simulink model "SPGF_FSK_0000_R2022b"  (R2022b)
settings: Solver=ode4  StartTime=0.0  StopTime=1.4  FixedStep=50e-6/50  RelTol=1e-3  EnableMultiTasking=on
undefined symbols (not defined in the file): D11, Delta
libraries: spsSeriesRLCBranchLib x1646, spsGroundLib x360, spsStairGeneratorLib x147, spsIdealSwitchLib x145, spsCurrentMeasurementLib x145, spsUniversalBridgeLib x76, spsThreePhaseSeriesRLCLoadLib x57, simulink x45, spsBistableLib x36, spsSequenceAnalyzerLib x31, spsThreePhaseParallelRLCLoadLib x20, spsThreePhaseTransformerTwoWindingsLib x20
(part 20 of 40)

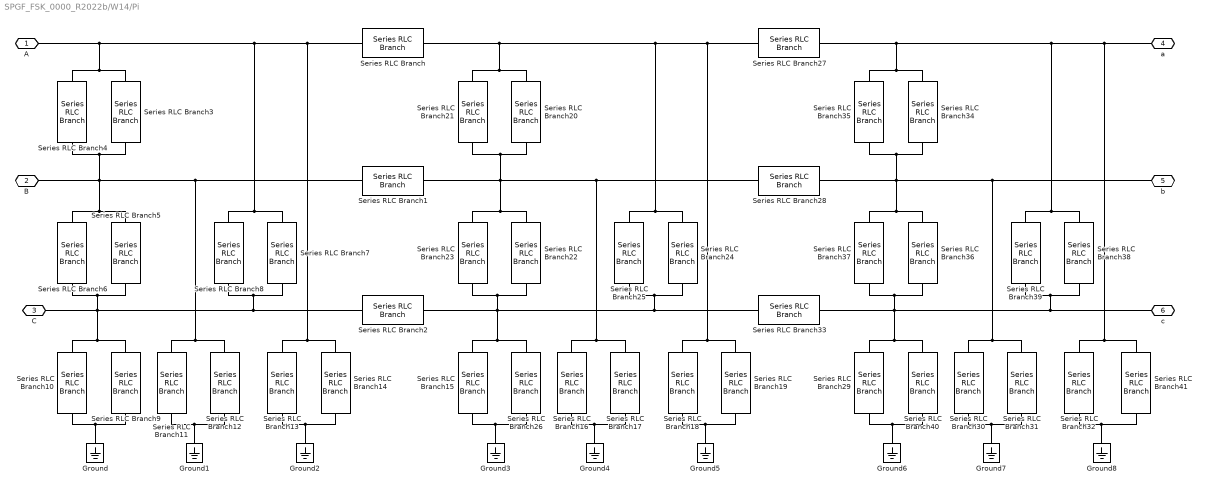
== system SPGF_FSK_0000_R2022b/W14/Pi ==
  Ground{,1..8} (9 alike) : spsGroundLib/Ground  LConnTagsString=a
  Series RLC Branch{,1..2,27..28,33} (6 alike) : spsSeriesRLCBranchLib/Series RLC Branch  LConnTagsString=__new0  RConnTagsString=__new0  BranchType=RL  Resistance=R/2  Inductance=L/2  SetiL0=off  InitialCurrent=0  Capacitance=1e-6  Setx0=off  InitialVoltage=0  Measurements=None
  Series RLC Branch{10..11,13,29..30,32} (6 alike) : spsSeriesRLCBranchLib/Series RLC Branch  LConnTagsString=__new0  RConnTagsString=__new0  BranchType=R  Resistance=Rfg*4  Inductance=L/2  SetiL0=off  InitialCurrent=0  Capacitance=1e-6  Setx0=off  InitialVoltage=0  Measurements=None
  Series RLC Branch{9,12,14,31,40..41} (6 alike) : spsSeriesRLCBranchLib/Series RLC Branch  LConnTagsString=__new0  RConnTagsString=__new0  BranchType=C  Resistance=R/2  Inductance=L/2  SetiL0=off  InitialCurrent=0  Capacitance=Cfg*0.25  Setx0=off  InitialVoltage=0  Measurements=None
  Series RLC Branch15 : spsSeriesRLCBranchLib/Series RLC Branch  LConnTagsString=__new0  RConnTagsString=__new0  BranchType=R  Resistance=Rfg*2  Inductance=L/2  SetiL0=off  InitialCurrent=0  Capacitance=1e-6  Setx0=off  InitialVoltage=0  Measurements=None
  Series RLC Branch16 : spsSeriesRLCBranchLib/Series RLC Branch  LConnTagsString=__new0  RConnTagsString=__new0  BranchType=R  Resistance=Rfg*2  Inductance=L/2  SetiL0=off  InitialCurrent=0  Capacitance=1e-6  Setx0=off  InitialVoltage=0  Measurements=None
  Series RLC Branch17 : spsSeriesRLCBranchLib/Series RLC Branch  LConnTagsString=__new0  RConnTagsString=__new0  BranchType=C  Resistance=R/2  Inductance=L/2  SetiL0=off  InitialCurrent=0  Capacitance=Cfg*0.5  Setx0=off  InitialVoltage=0  Measurements=None
  Series RLC Branch18 : spsSeriesRLCBranchLib/Series RLC Branch  LConnTagsString=__new0  RConnTagsString=__new0  BranchType=R  Resistance=Rfg*2  Inductance=L/2  SetiL0=off  InitialCurrent=0  Capacitance=1e-6  Setx0=off  InitialVoltage=0  Measurements=None
  Series RLC Branch19 : spsSeriesRLCBranchLib/Series RLC Branch  LConnTagsString=__new0  RConnTagsString=__new0  BranchType=C  Resistance=R/2  Inductance=L/2  SetiL0=off  InitialCurrent=0  Capacitance=Cfg*0.5  Setx0=off  InitialVoltage=0  Measurements=None
  Series RLC Branch20 : spsSeriesRLCBranchLib/Series RLC Branch  LConnTagsString=__new0  RConnTagsString=__new0  BranchType=C  Resistance=R/2  Inductance=L/2  SetiL0=off  InitialCurrent=0  Capacitance=Cmf*0.5  Setx0=off  InitialVoltage=0  Measurements=None
  Series RLC Branch21 : spsSeriesRLCBranchLib/Series RLC Branch  LConnTagsString=__new0  RConnTagsString=__new0  BranchType=R  Resistance=Rmf*2  Inductance=L/2  SetiL0=off  InitialCurrent=0  Capacitance=1e-6  Setx0=off  InitialVoltage=0  Measurements=None
  Series RLC Branch22 : spsSeriesRLCBranchLib/Series RLC Branch  LConnTagsString=__new0  RConnTagsString=__new0  BranchType=C  Resistance=R/2  Inductance=L/2  SetiL0=off  InitialCurrent=0  Capacitance=Cmf*0.5  Setx0=off  InitialVoltage=0  Measurements=None
  Series RLC Branch23 : spsSeriesRLCBranchLib/Series RLC Branch  LConnTagsString=__new0  RConnTagsString=__new0  BranchType=R  Resistance=Rmf*2  Inductance=L/2  SetiL0=off  InitialCurrent=0  Capacitance=1e-6  Setx0=off  InitialVoltage=0  Measurements=None
  Series RLC Branch24 : spsSeriesRLCBranchLib/Series RLC Branch  LConnTagsString=__new0  RConnTagsString=__new0  BranchType=C  Resistance=R/2  Inductance=L/2  SetiL0=off  InitialCurrent=0  Capacitance=Cmf*0.5  Setx0=off  InitialVoltage=0  Measurements=None
  Series RLC Branch25 : spsSeriesRLCBranchLib/Series RLC Branch  LConnTagsString=__new0  RConnTagsString=__new0  BranchType=R  Resistance=Rmf*2  Inductance=L/2  SetiL0=off  InitialCurrent=0  Capacitance=1e-6  Setx0=off  InitialVoltage=0  Measurements=None
  Series RLC Branch26 : spsSeriesRLCBranchLib/Series RLC Branch  LConnTagsString=__new0  RConnTagsString=__new0  BranchType=C  Resistance=R/2  Inductance=L/2  SetiL0=off  InitialCurrent=0  Capacitance=Cfg*0.5  Setx0=off  InitialVoltage=0  Measurements=None
  Series RLC Branch{3,5,7,34,36,38} (6 alike) : spsSeriesRLCBranchLib/Series RLC Branch  LConnTagsString=__new0  RConnTagsString=__new0  BranchType=C  Resistance=R/2  Inductance=L/2  SetiL0=off  InitialCurrent=0  Capacitance=Cmf*0.25  Setx0=off  InitialVoltage=0  Measurements=None
  Series RLC Branch{4,6,8,35,37,39} (6 alike) : spsSeriesRLCBranchLib/Series RLC Branch  LConnTagsString=__new0  RConnTagsString=__new0  BranchType=R  Resistance=Rmf*4  Inductance=L/2  SetiL0=off  InitialCurrent=0  Capacitance=1e-6  Setx0=off  InitialVoltage=0  Measurements=None
  A : PMIOPort  Side=Left
  B : PMIOPort  Port=2  Side=Left
  C : PMIOPort  Port=3  Side=Left
  a : PMIOPort  Port=4  Side=Right
  b : PMIOPort  Port=5  Side=Right
  c : PMIOPort  Port=6  Side=Right
  connections:
  Ground8/LConn1 -- Series RLC Branch41/RConn1 -- Series RLC Branch32/RConn1
  Ground7/LConn1 -- Series RLC Branch30/RConn1 -- Series RLC Branch31/RConn1
  Ground6/LConn1 -- Series RLC Branch40/RConn1 -- Series RLC Branch29/RConn1
  Series RLC Branch40/LConn1 -- Series RLC Branch33/RConn1 -- Series RLC Branch38/RConn1 -- Series RLC Branch39/RConn1 -- c/RConn1 -- Series RLC Branch37/RConn1 -- Series RLC Branch36/RConn1 -- Series RLC Branch29/LConn1
  Series RLC Branch35/LConn1 -- Series RLC Branch27/RConn1 -- Series RLC Branch39/LConn1 -- Series RLC Branch38/LConn1 -- Series RLC Branch32/LConn1 -- Series RLC Branch41/LConn1 -- a/RConn1 -- Series RLC Branch34/LConn1
  Series RLC Branch30/LConn1 -- Series RLC Branch28/RConn1 -- Series RLC Branch37/LConn1 -- Series RLC Branch36/LConn1 -- Series RLC Branch34/RConn1 -- Series RLC Branch35/RConn1 -- b/RConn1 -- Series RLC Branch31/LConn1
  Series RLC Branch19/RConn1 -- Series RLC Branch18/RConn1 -- Ground5/LConn1
  Series RLC Branch16/RConn1 -- Series RLC Branch17/RConn1 -- Ground4/LConn1
  Ground3/LConn1 -- Series RLC Branch15/RConn1 -- Series RLC Branch26/RConn1
  Series RLC Branch23/RConn1 -- Series RLC Branch22/RConn1 -- Series RLC Branch24/RConn1 -- Series RLC Branch25/RConn1 -- Series RLC Branch33/LConn1 -- Series RLC Branch2/RConn1 -- Series RLC Branch15/LConn1 -- Series RLC Branch26/LConn1
  Series RLC Branch25/LConn1 -- Series RLC Branch24/LConn1 -- Series RLC Branch18/LConn1 -- Series RLC Branch19/LConn1 -- Series RLC Branch27/LConn1 -- Series RLC Branch/RConn1 -- Series RLC Branch20/LConn1 -- Series RLC Branch21/LConn1
  Series RLC Branch21/RConn1 -- Series RLC Branch20/RConn1 -- Series RLC Branch22/LConn1 -- Series RLC Branch23/LConn1 -- Series RLC Branch1/RConn1 -- Series RLC Branch28/LConn1 -- Series RLC Branch16/LConn1 -- Series RLC Branch17/LConn1
  Ground2/LConn1 -- Series RLC Branch14/RConn1 -- Series RLC Branch13/RConn1
  Ground1/LConn1 -- Series RLC Branch11/RConn1 -- Series RLC Branch12/RConn1
  Series RLC Branch10/RConn1 -- Ground/LConn1 -- Series RLC Branch9/RConn1
  Series RLC Branch10/LConn1 -- Series RLC Branch6/RConn1 -- Series RLC Branch5/RConn1 -- C/RConn1 -- Series RLC Branch7/RConn1 -- Series RLC Branch8/RConn1 -- Series RLC Branch2/LConn1 -- Series RLC Branch9/LConn1
  Series RLC Branch14/LConn1 -- Series RLC Branch/LConn1 -- Series RLC Branch8/LConn1 -- Series RLC Branch7/LConn1 -- Series RLC Branch3/LConn1 -- Series RLC Branch4/LConn1 -- A/RConn1 -- Series RLC Branch13/LConn1
  Series RLC Branch1/LConn1 -- Series RLC Branch3/RConn1 -- Series RLC Branch4/RConn1 -- B/RConn1 -- Series RLC Branch6/LConn1 -- Series RLC Branch5/LConn1 -- Series RLC Branch11/LConn1 -- Series RLC Branch12/LConn1

== system SPGF_FSK_0000_R2022b/W14/Q ==
  breaker : Subsystem  Commented=on  mask{SwitchA=off, SwitchB=off, SwitchC=off, InitialStatus=[1 1 1], BreakerResistance=0.0001, SnubberResistance=1e6, SnubberCapacitance=inf, TransitionTimes=[0.5 0.7], ShiftTimes=[0 0 0]}
      mask prompts: SwitchA "Switching of phase A"; SwitchB "Switching of phase B"; SwitchC "Switching of phase C"; InitialStatus "Initial status of phase breaker [A, B, C]"; BreakerResistance "Breaker resistance Ron (ohms) :"; SnubberResistance "Snubbers resistance Rp (ohms) :"; SnubberCapacitance "Snubbers capacitance Cp (F) :"; TransitionTimes "Transition times (s) :"; ShiftTimes "Time differences for switch [tA, tB, tC] (s) :"
      mask init: same as SPGF_FSK_0000_R2022b/Feed/Q/breaker
      mask Display:
      | % port_label('input',1,'Iabc');
      | 
      | port_label('lconn',1,'A');
      | port_label('lconn',2,'B');
      | port_label('lconn',3,'C');
      | 
      | port_label('rconn',1,'a');
      | port_label('rconn',2,'b');
      | port_label('rconn',3,'c');
      | 
      | disp('   Q    ');
  meas : Subsystem
  shunt : Subsystem
  A : PMIOPort  Side=Right
  B : PMIOPort  Port=2  Side=Right
  C : PMIOPort  Port=3  Side=Right
  a : PMIOPort  Port=4  Side=Left
  b : PMIOPort  Port=5  Side=Left
  c : PMIOPort  Port=6  Side=Left
  connections:
  shunt/LConn3 -- C/RConn1 -- breaker/LConn3
  shunt/LConn2 -- B/RConn1 -- breaker/LConn2
  A/RConn1 -- shunt/LConn1 -- breaker/LConn1
  meas/RConn1 -- a/RConn1
  meas/RConn2 -- b/RConn1
  meas/RConn3 -- c/RConn1
  meas/LConn3 -- breaker/RConn3 -- shunt/RConn3
  meas/LConn2 -- breaker/RConn2 -- shunt/RConn2
  meas/LConn1 -- breaker/RConn1 -- shunt/RConn1

== system SPGF_FSK_0000_R2022b/W14/concentrated ==
  Ccs/1 : spsSeriesRLCBranchLib/Series RLC Branch  LConnTagsString=__new0  RConnTagsString=__new0  BranchType=C  Resistance=190  Inductance=1e-3  SetiL0=off  InitialCurrent=0  Capacitance=-C_matrix(1,2)/2  Setx0=off  InitialVoltage=0  Measurements=None
  Ccs/2 : spsSeriesRLCBranchLib/Series RLC Branch  LConnTagsString=__new0  RConnTagsString=__new0  BranchType=C  Resistance=190  Inductance=1e-3  SetiL0=off  InitialCurrent=0  Capacitance=-C_matrix(1,2)/2  Setx0=off  InitialVoltage=0  Measurements=None
  Ccs2/1 : spsSeriesRLCBranchLib/Series RLC Branch  LConnTagsString=__new0  RConnTagsString=__new0  BranchType=C  Resistance=190  Inductance=1e-3  SetiL0=off  InitialCurrent=0  Capacitance=-C_matrix(3,4)/2  Setx0=off  InitialVoltage=0  Measurements=None
  Ccs2/2 : spsSeriesRLCBranchLib/Series RLC Branch  LConnTagsString=__new0  RConnTagsString=__new0  BranchType=C  Resistance=190  Inductance=1e-3  SetiL0=off  InitialCurrent=0  Capacitance=-C_matrix(3,4)/2  Setx0=off  InitialVoltage=0  Measurements=None
  Ccs2/3 : spsSeriesRLCBranchLib/Series RLC Branch  LConnTagsString=__new0  RConnTagsString=__new0  BranchType=R  Resistance=-Rg_matrix(3,4)*2  Inductance=1e-3  SetiL0=off  InitialCurrent=0  Capacitance=Rg_matrix(3,4)*2  Setx0=off  InitialVoltage=0  Measurements=None
  Ccs2/4 : spsSeriesRLCBranchLib/Series RLC Branch  LConnTagsString=__new0  RConnTagsString=__new0  BranchType=R  Resistance=-Rg_matrix(3,4)*2  Inductance=1e-3  SetiL0=off  InitialCurrent=0  Capacitance=Rg_matrix(3,4)*2  Setx0=off  InitialVoltage=0  Measurements=None
  Ccs3/1 : spsSeriesRLCBranchLib/Series RLC Branch  LConnTagsString=__new0  RConnTagsString=__new0  BranchType=C  Resistance=190  Inductance=1e-3  SetiL0=off  InitialCurrent=0  Capacitance=-C_matrix(5,6)/2  Setx0=off  InitialVoltage=0  Measurements=None
  Ccs3/2 : spsSeriesRLCBranchLib/Series RLC Branch  LConnTagsString=__new0  RConnTagsString=__new0  BranchType=C  Resistance=190  Inductance=1e-3  SetiL0=off  InitialCurrent=0  Capacitance=-C_matrix(5,6)/2  Setx0=off  InitialVoltage=0  Measurements=None
  Ccs3/3 : spsSeriesRLCBranchLib/Series RLC Branch  LConnTagsString=__new0  RConnTagsString=__new0  BranchType=R  Resistance=-Rg_matrix(5,6)*2  Inductance=1e-3  SetiL0=off  InitialCurrent=0  Capacitance=-C_matrix(5,6)/2  Setx0=off  InitialVoltage=0  Measurements=None
  Ccs3/4 : spsSeriesRLCBranchLib/Series RLC Branch  LConnTagsString=__new0  RConnTagsString=__new0  BranchType=R  Resistance=-Rg_matrix(5,6)*2  Inductance=1e-3  SetiL0=off  InitialCurrent=0  Capacitance=-C_matrix(5,6)/2  Setx0=off  InitialVoltage=0  Measurements=None
  Csg/2 : spsSeriesRLCBranchLib/Series RLC Branch  LConnTagsString=__new0  RConnTagsString=__new0  BranchType=C  Resistance=190  Inductance=1e-3  SetiL0=off  InitialCurrent=0  Capacitance=( C_matrix(1,2) + C_matrix(2,2) )/2  Setx0=off  InitialVoltage=0  Measurements=None
  Csg1/1 : spsSeriesRLCBranchLib/Series RLC Branch  LConnTagsString=__new0  RConnTagsString=__new0  BranchType=C  Resistance=190  Inductance=1e-3  SetiL0=off  InitialCurrent=0  Capacitance=( C_matrix(1,2) + C_matrix(2,2) )/2  Setx0=off  InitialVoltage=0  Measurements=None
  Csg2/1 : spsSeriesRLCBranchLib/Series RLC Branch  LConnTagsString=__new0  RConnTagsString=__new0  BranchType=C  Resistance=190  Inductance=1e-3  SetiL0=off  InitialCurrent=0  Capacitance=( C_matrix(3,4) + C_matrix(4,4) )/2  Setx0=off  InitialVoltage=0  Measurements=None
  Csg2/2 : spsSeriesRLCBranchLib/Series RLC Branch  LConnTagsString=__new0  RConnTagsString=__new0  BranchType=C  Resistance=190  Inductance=1e-3  SetiL0=off  InitialCurrent=0  Capacitance=( C_matrix(3,4) + C_matrix(4,4) )/2  Setx0=off  InitialVoltage=0  Measurements=None
  Csg3/1 : spsSeriesRLCBranchLib/Series RLC Branch  LConnTagsString=__new0  RConnTagsString=__new0  BranchType=C  Resistance=190  Inductance=1e-3  SetiL0=off  InitialCurrent=0  Capacitance=( C_matrix(5,6) + C_matrix(6,6) ) /2  Setx0=off  InitialVoltage=0  Measurements=None
  Csg3/2 : spsSeriesRLCBranchLib/Series RLC Branch  LConnTagsString=__new0  RConnTagsString=__new0  BranchType=C  Resistance=190  Inductance=1e-3  SetiL0=off  InitialCurrent=0  Capacitance=( C_matrix(5,6) + C_matrix(6,6) ) /2  Setx0=off  InitialVoltage=0  Measurements=None
  Ground{1..4} (4 alike) : spsGroundLib/Ground  LConnTagsString=a
  RL : spsMutualInductanceLib/Mutual Inductance  LConnTagsString=a|b|c|L4|L5|L6  RConnTagsString=A|B|C|R4|R5|R6  TypeOfMutual=Generalized mutual inductance  NumberOfWindings=6  SelfImpedance1=[1.1 1.1e-03]  SelfImpedance2=[ 1.1 1.1e-03]  ThreeWindings=on  SelfImpedance3=[ 1.1 1.1e-03]  MutualImpedance=[1.0 1.0e-03]  InductanceMatrix=L_matrix  ResistanceMatrix=R_matrix  Measurements=None
      settings: LibrarySourceBlock=sps_lib/Passives/Mutual Inductance
  Rcs*2 : spsSeriesRLCBranchLib/Series RLC Branch  LConnTagsString=__new0  RConnTagsString=__new0  BranchType=R  Resistance=-Rg_matrix(1,2)*2  Inductance=1e-3  SetiL0=off  InitialCurrent=0  Capacitance=Rg_matrix(1,2)*2  Setx0=off  InitialVoltage=0  Measurements=None
  Rgcs1/1 : spsSeriesRLCBranchLib/Series RLC Branch  LConnTagsString=__new0  RConnTagsString=__new0  BranchType=R  Resistance=-Rg_matrix(1,2)*2  Inductance=1e-3  SetiL0=off  InitialCurrent=0  Capacitance=Rg_matrix(1,2)*2  Setx0=off  InitialVoltage=0  Measurements=None
  Rgsg1/1 : spsSeriesRLCBranchLib/Series RLC Branch  LConnTagsString=__new0  RConnTagsString=__new0  BranchType=R  Resistance=(Rg_matrix(4,4)+Rg_matrix(3,4))*2  Inductance=1e-3  SetiL0=off  InitialCurrent=0  Capacitance=Rg_matrix(1,2)*2  Setx0=off  InitialVoltage=0  Measurements=None
  Rgsg1/2 : spsSeriesRLCBranchLib/Series RLC Branch  LConnTagsString=__new0  RConnTagsString=__new0  BranchType=R  Resistance=(Rg_matrix(2,2)+Rg_matrix(1,2))*2  Inductance=1e-3  SetiL0=off  InitialCurrent=0  Capacitance=Rg_matrix(1,2)*2  Setx0=off  InitialVoltage=0  Measurements=None
  Rgsg1/3 : spsSeriesRLCBranchLib/Series RLC Branch  LConnTagsString=__new0  RConnTagsString=__new0  BranchType=R  Resistance=(Rg_matrix(4,4)+Rg_matrix(3,4))*2  Inductance=1e-3  SetiL0=off  InitialCurrent=0  Capacitance=Rg_matrix(1,2)*2  Setx0=off  InitialVoltage=0  Measurements=None
  Rgsg1/4 : spsSeriesRLCBranchLib/Series RLC Branch  LConnTagsString=__new0  RConnTagsString=__new0  BranchType=R  Resistance=(Rg_matrix(2,2)+Rg_matrix(1,2))*2  Inductance=1e-3  SetiL0=off  InitialCurrent=0  Capacitance=Rg_matrix(1,2)*2  Setx0=off  InitialVoltage=0  Measurements=None
  Rsg*2 : spsSeriesRLCBranchLib/Series RLC Branch  LConnTagsString=__new0  RConnTagsString=__new0  BranchType=R  Resistance=(Rg_matrix(6,6)+Rg_matrix(5,6))*2  Inductance=1e-3  SetiL0=off  InitialCurrent=0  Capacitance=Rg_matrix(1,2)*2  Setx0=off  InitialVoltage=0  Measurements=None
  Rsg1/1 : spsSeriesRLCBranchLib/Series RLC Branch  LConnTagsString=__new0  RConnTagsString=__new0  BranchType=R  Resistance=(Rg_matrix(6,6)+Rg_matrix(5,6))*2  Inductance=1e-3  SetiL0=off  InitialCurrent=0  Capacitance=Rg_matrix(1,2)*2  Setx0=off  InitialVoltage=0  Measurements=None
  A : PMIOPort  Side=Left
  B : PMIOPort  Port=2  Side=Left
  C : PMIOPort  Port=3  Side=Left
  a : PMIOPort  Port=4  Side=Right
  b : PMIOPort  Port=5  Side=Right
  c : PMIOPort  Port=6  Side=Right
  connections:
  RL/LConn6 -- Ground3/LConn1 -- Rgsg1/2/LConn1 -- Csg/2/LConn1 -- Rcs*2/LConn1 -- Ccs/2/LConn1 -- RL/LConn2 -- RL/LConn4 -- Rgsg1/1/LConn1 -- Csg2/2/LConn1 -- Ccs2/3/LConn1 -- Ccs2/2/LConn1 -- Rsg*2/LConn1 -- Csg3/2/LConn1 -- Ccs3/3/LConn1 -- Ccs3/2/LConn1
  Rsg1/1/RConn1 -- Rgsg1/3/RConn1 -- Rgsg1/4/RConn1 -- Csg3/1/RConn1 -- Csg2/1/RConn1 -- Ground2/LConn1 -- Csg1/1/RConn1
  Rgsg1/3/LConn1 -- Ccs2/4/LConn1 -- Csg2/1/LConn1 -- Ccs2/1/LConn1 -- RL/RConn4 -- Rgsg1/4/LConn1 -- Rgcs1/1/LConn1 -- Csg1/1/LConn1 -- Ccs/1/LConn1 -- RL/RConn2 -- Ground4/LConn1 -- RL/RConn6 -- Ccs3/1/LConn1 -- Rsg1/1/LConn1 -- Ccs3/4/LConn1 -- Csg3/1/LConn1
  Rsg*2/RConn1 -- Rgsg1/1/RConn1 -- Rgsg1/2/RConn1 -- Csg3/2/RConn1 -- Csg2/2/RConn1 -- Ground1/LConn1 -- Csg/2/RConn1
  a/RConn1 -- RL/RConn1 -- Rgcs1/1/RConn1 -- Ccs/1/RConn1
  b/RConn1 -- RL/RConn3 -- Ccs2/4/RConn1 -- Ccs2/1/RConn1
  Ccs3/1/RConn1 -- c/RConn1 -- RL/RConn5 -- Ccs3/4/RConn1
  RL/LConn1 -- A/RConn1 -- Rcs*2/RConn1 -- Ccs/2/RConn1
  RL/LConn3 -- B/RConn1 -- Ccs2/3/RConn1 -- Ccs2/2/RConn1
  Ccs3/2/RConn1 -- C/RConn1 -- RL/LConn5 -- Ccs3/3/RConn1

== system SPGF_FSK_0000_R2022b/W15/DPL ==
  Ccs2/1 : spsSeriesRLCBranchLib/Series RLC Branch  LConnTagsString=__new0  RConnTagsString=__new0  BranchType=R  Resistance=-Rg_matrix(3,4)*2  Inductance=1e-3  SetiL0=off  InitialCurrent=0  Capacitance=Rg_matrix(3,4)*2  Setx0=off  InitialVoltage=0  Measurements=None
  Ccs2/3 : spsSeriesRLCBranchLib/Series RLC Branch  LConnTagsString=__new0  RConnTagsString=__new0  BranchType=R  Resistance=-Rg_matrix(3,4)*2  Inductance=1e-3  SetiL0=off  InitialCurrent=0  Capacitance=Rg_matrix(3,4)*2  Setx0=off  InitialVoltage=0  Measurements=None
  Ccs3/1 : spsSeriesRLCBranchLib/Series RLC Branch  LConnTagsString=__new0  RConnTagsString=__new0  BranchType=R  Resistance=-Rg_matrix(5,6)*2  Inductance=1e-3  SetiL0=off  InitialCurrent=0  Capacitance=-C_matrix(5,6)/2  Setx0=off  InitialVoltage=0  Measurements=None
  Ccs3/3 : spsSeriesRLCBranchLib/Series RLC Branch  LConnTagsString=__new0  RConnTagsString=__new0  BranchType=R  Resistance=-Rg_matrix(5,6)*2  Inductance=1e-3  SetiL0=off  InitialCurrent=0  Capacitance=-C_matrix(5,6)/2  Setx0=off  InitialVoltage=0  Measurements=None
  DPL : spsDistributedParametersLineLib/Distributed Parameters Line  Phases=6  Length=LineLength  Frequency=Frequency  Resistance=R_matrix  Inductance=L_matrix  Capacitance=C_matrix  x1=[-1.75e-05 -0.970054197486436 4562.89829084074 0 -2575.25598522641 0 -4598.44133827164;-1.7e-05 -0.970312885821604 4564.17604930488 0 -2575.97713983532 0 -4598.03326492144;-1.65e-05 -0.97057155021526 4565.45369515248 0 -2576.69823088453 0 -4597.62507811931;-1.6e-05 -0.970830190661023 4566.73122835204 0 -2577.41925835626 0 -4597.21677787533;-1.55e-05 -0.971088807152512 4568.00864887201 0 -2578.14022223273 0 -4596.80836419957;-1.5e-05 -0.971347399683345 4569.28595668089 0 -2578.86112249613 0 -4596.39983710211;-1.45e-05 -0.971605968247141 4570.56315174716 0 -2579.58195912868 0 -4595.99119659304;-1.4e-05 -0.971864512837521 4571.84023403931 0 -2580.3027321126 0 -4595.58244268242;-1.35e-05 -0.972123033448105 4573.11720352581 0 -2581.02344143011 0 -4595.17357538036;-1.3e-05 -0.972381530072515 4574.39406017518 0 -2581.74408706341 0 -4594.76459469693;-1.25e-05 -0.972640002704373 4575.67080395589 0 -2582.46466899473 0 -4594.35550064223;-1.2e-05 -0.9728984513373 4576.94743483645 0 -2583.18518720629 0 -4593.94629322635;-1.15e-05 -0.973156875964921 4578.22395278537 0 -2583.90564168031 0 -4593.53697245939;-1.1e-05 -0.973415276580858 4579.50035777113 0 -2584.62603239901 0 -4593.12753835145;-1.05e-05 -0.973673653178736 4580.77664976225 0 -2585.34635934462 0 -4592.71799091263;-1e-05 -0.973932005752179 4582.05282872724 0 -2586.06662249937 0 -4592.30833015303;-9.5e-06 -0.974190334294813 4583.32889463461 0 -2586.78682184548 0 -4591.89855608277;-9e-06 -0.974448638800265 4584.60484745287 0 -2587.50695736519 0 -4591.48866871195;-8.5e-06 -0.97470691926216 4585.88068715053 0 -2588.22702904072 0 -4591.0786680507;-8e-06 -0.974965175674126 4587.15641369613 0 -2588.94703685431 0 -4590.66855410911;-7.5e-06 -0.97522340802979 4588.43202705819 0 -2589.66698078819 0 -4590.25832689732;-7e-06 -0.975481616322782 4589.70752720521 0 -2590.3868608246 0 -4589.84798642545;-6.5e-06 -0.975739800546729 4590.98291410575 0 -2591.10667694577 0 -4589.43753270362;-6e-06 -0.975997960695262 4592.25818772832 0 -2591.82642913395 0 -4589.02696574195;-5.5e-06 -0.97625609676201 4593.53334804147 0 -2592.54611737138 0 -4588.61628555059;-5e-06 -0.976514208740605 4594.80839501372 0 -2593.2657416403 0 -4588.20549213965;-4.5e-06 -0.976772296624677 4596.08332861362 0 -2593.98530192295 0 -4587.79458551928;-4e-06 -0.977030360407859 4597.35814880971 -12.2435730185773 -2594.70479820157 0 -4587.38356569962;-3.5e-06 -0.977288400083784 4598.63285557053 -12.2467162601887 -2595.42423045843 0 -4586.97243269081;-3e-06 -0.977546415646083 4599.90744886464 -12.2498591996244 -2596.14359867575 0 -4586.56118650299;-2.5e-06 -0.977804407088392 4601.18192866058 -12.253001836807 -2596.8629028358 -8123.40722149064 -4586.1498271463;-2e-06 -0.978062374404344 4602.4562949269 -12.2561441716589 -2597.58214292083 -8122.67838381002 -4585.73835463091;-1.5e-06 -0.978320317587574 4603.73054763217 -12.2592862041026 -2598.30131891309 -8121.94934571034 -4585.32676896696;-1e-06 -0.978578236631719 4605.00468674494 -12.2624279340604 -2599.02043079483 -8121.2201072096 -4584.9150701646;-5e-07 -0.978836131530412 4606.27871223378 -12.2655693614551 -2599.73947854831 -8120.49066832578 -4584.503258234]  x2=[-1.75e-05 -0.969909174189962 4563.53149309113 0 -2575.61335849667 0 -4603.35101620542;-1.7e-05 -0.97016841316058 4564.8106332212 0 -2576.33529290456 0 -4602.94292906916;-1.65e-05 -0.970427628193253 4566.08966071909 0 -2577.05716374393 0 -4602.53472835983;-1.6e-05 -0.970686819281583 4567.36857555322 0 -2577.77897099696 0 -4602.12641408751;-1.55e-05 -0.970945986419177 4568.64737769206 0 -2578.50071464584 0 -4601.71798626227;-1.5e-05 -0.971205129599638 4569.92606710404 0 -2579.22239467276 0 -4601.30944489419;-1.45e-05 -0.971464248816574 4571.20464375762 0 -2579.94401105993 0 -4600.90078999336;-1.4e-05 -0.97172334406359 4572.48310762124 0 -2580.66556378953 0 -4600.49202156984;-1.35e-05 -0.971982415334293 4573.76145866336 0 -2581.38705284376 0 -4600.08313963374;-1.3e-05 -0.972241462622292 4575.03969685245 0 -2582.10847820481 0 -4599.67414419513;-1.25e-05 -0.972500485921194 4576.31782215695 0 -2582.8298398549 0 -4599.26503526412;-1.2e-05 -0.972759485224609 4577.59583454534 0 -2583.55113777621 0 -4598.85581285079;-1.15e-05 -0.973018460526145 4578.87373398608 0 -2584.27237195095 0 -4598.44647696524;-1.1e-05 -0.973277411819413 4580.15152044763 0 -2584.99354236133 0 -4598.03702761757;-1.05e-05 -0.973536339098024 4581.42919389848 0 -2585.71464898955 0 -4597.62746481788;-1e-05 -0.973795242355589 4582.7067543071 0 -2586.43569181781 0 -4597.21778857629;-9.5e-06 -0.974054121585719 4583.98420164195 0 -2587.15667082834 0 -4596.80799890289;-9e-06 -0.974312976782026 4585.26153587154 0 -2587.87758600333 0 -4596.3980958078;-8.5e-06 -0.974571807938125 4586.53875696432 0 -2588.598437325 0 -4595.98807930114;-8e-06 -0.974830615047629 4587.81586488881 0 -2589.31922477557 0 -4595.57794939301;-7.5e-06 -0.975089398104151 4589.09285961347 0 -2590.03994833724 0 -4595.16770609354;-7e-06 -0.975348157101307 4590.3697411068 0 -2590.76060799224 0 -4594.75734941286;-6.5e-06 -0.975606892032711 4591.6465093373 0 -2591.48120372279 0 -4594.34687936108;-6e-06 -0.975865602891981 4592.92316427347 0 -2592.2017355111 0 -4593.93629594834;-5.5e-06 -0.976124289672731 4594.1997058838 0 -2592.9222033394 0 -4593.52559918476;-5e-06 -0.976382952368581 4595.47613413679 0 -2593.6426071899 0 -4593.11478908048;-4.5e-06 -0.976641590973146 4596.75244900096 0 -2594.36294704484 0 -4592.70386564564;-4e-06 -0.976900205480047 4598.0286504448 -12.2400263625723 -2595.08322288644 0 -4592.29282889037;-3.5e-06 -0.977158795882901 4599.30473843684 -12.2431783125652 -2595.80343469693 0 -4591.88167882482;-3e-06 -0.977417362175328 4600.58071294558 -12.2463299604697 -2596.52358245853 0 -4591.47041545913;-2.5e-06 -0.977675904350949 4601.85657393954 -12.2494813062082 -2597.24366615349 -8132.10286531618 -4591.05903880345;-2e-06 -0.977934422403383 4603.13232138724 -12.2526323497029 -2597.96368576402 -8131.37399677944 -4590.64754886792;-1.5e-06 -0.978192916326253 4604.40795525721 -12.255783090876 -2598.68364127237 -8130.64492760909 -4590.23594566271;-1e-06 -0.97845138611318 4605.68347551796 -12.2589335296497 -2599.40353266077 -8129.91565782311 -4589.82422919797;-5e-07 -0.978709831757787 4606.95888213803 -12.2620836659464 -2600.12335991146 -8129.1861874395 -4589.41239948385]  x3=[-1.75e-05 -0.00229496214449278 43.4939554001372 0 -181.870549246955 0 -363.640879762457;-1.7e-05 -0.00229664365019055 43.5123375348381 0 -181.923927171716 0 -363.610096045722;-1.65e-05 -0.00229832509922091 43.5307185959151 0 -181.977300607684 0 -363.579303357267;-1.6e-05 -0.00230000649154237 43.5490985829147 0 -182.030669553542 0 -363.548501697852;-1.55e-05 -0.00230168782711345 43.5674774953834 0 -182.084034007974 0 -363.517691068237;-1.5e-05 -0.00230336910589265 43.5858553328677 0 -182.137393969662 0 -363.486871469183;-1.45e-05 -0.0023050503278385 43.6042320949141 0 -182.19074943729 0 -363.456042901451;-1.4e-05 -0.00230673149290952 43.6226077810692 0 -182.244100409541 0 -363.425205365799;-1.35e-05 -0.00230841260106421 43.6409823908796 0 -182.297446885099 0 -363.39435886299;-1.3e-05 -0.00231009365226111 43.6593559238919 0 -182.350788862649 0 -363.363503393785;-1.25e-05 -0.00231177464645873 43.6777283796527 0 -182.404126340872 0 -363.332638958945;-1.2e-05 -0.0023134555836156 43.6960997577089 0 -182.457459318455 0 -363.301765559231;-1.15e-05 -0.00231513646369024 43.714470057607 0 -182.51078779408 0 -363.270883195405;-1.1e-05 -0.00231681728664118 43.7328392788937 0 -182.564111766432 0 -363.23999186823;-1.05e-05 -0.00231849805242694 43.751207421116 0 -182.617431234195 0 -363.209091578467;-1e-05 -0.00232017876100606 43.7695744838204 0 -182.670746196053 0 -363.178182326879;-9.5e-06 -0.00232185941233706 43.7879404665539 0 -182.724056650692 0 -363.147264114229;-9e-06 -0.00232354000637847 43.8063053688633 0 -182.777362596795 0 -363.116336941279;-8.5e-06 -0.00232522054308884 43.8246691902954 0 -182.830664033048 0 -363.085400808793;-8e-06 -0.00232690102242668 43.8430319303971 0 -182.883960958134 0 -363.054455717533;-7.5e-06 -0.00232858144435055 43.8613935887154 0 -182.93725337074 0 -363.023501668264;-7e-06 -0.00233026180881897 43.8797541647972 0 -182.99054126955 0 -362.992538661749;-6.5e-06 -0.00233194211579048 43.8981136581895 0 -183.04382465325 0 -362.961566698752;-6e-06 -0.00233362236522363 43.9164720684392 0 -183.097103520524 0 -362.930585780037;-5.5e-06 -0.00233530255707696 43.9348293950934 0 -183.150377870058 0 -362.899595906369;-5e-06 -0.00233698269130901 43.9531856376991 0 -183.203647700538 0 -362.868597078513;-4.5e-06 -0.00233866276787832 43.9715407958035 0 -183.256913010649 0 -362.837589297233;-4e-06 -0.00234034278674344 43.9898948689536 -0.568519302327501 -183.310173799076 0 -362.806572563294;-3.5e-06 -0.00234202274786291 44.0082478566965 -0.568702120753468 -183.363430064507 0 -362.775546877462;-3e-06 -0.00234370265119529 44.0265997585794 -0.568884925147273 -183.416681805626 0 -362.744512240502;-2.5e-06 -0.00234538249669913 44.0449505741496 -0.569067715504404 -183.46992902112 -132.458542183644 -362.713468653179;-2e-06 -0.00234706228433297 44.0633003029541 -0.569250491820353 -183.523171709675 -132.450102121752 -362.682416116261;-1.5e-06 -0.00234874201405537 44.0816489445403 -0.569433254090608 -183.576409869978 -132.441658791785 -362.651354630513;-1e-06 -0.00235042168582488 44.0999964984554 -0.569616002310662 -183.629643500714 -132.433212193951 -362.620284196702;-5e-07 -0.00235210129960007 44.1183429642467 -0.569798736476004 -183.68287260057 -132.424762328459 -362.589204815593]  x4=[-1.75e-05 -0.00894965597000911 55.5920439086836 0 -180.906113194492 0 -332.202894343638;-1.7e-05 -0.00895099537290878 55.6014516647724 0 -180.954480230298 0 -332.172020395278;-1.65e-05 -0.00895233455495151 55.6108580489503 0 -181.002842801231 0 -332.141138250902;-1.6e-05 -0.00895367351610423 55.6202630609854 0 -181.051200906098 0 -332.110247911272;-1.55e-05 -0.00895501225633391 55.6296667006454 0 -181.099554543705 0 -332.07934937715;-1.5e-05 -0.00895635077560752 55.6390689676985 0 -181.147903712861 0 -332.048442649298;-1.45e-05 -0.00895768907389203 55.6484698619125 0 -181.19624841237 0 -332.01752772848;-1.4e-05 -0.00895902715115443 55.6578693830556 0 -181.244588641042 0 -331.986604615457;-1.35e-05 -0.00896036500736169 55.6672675308959 0 -181.292924397683 0 -331.955673310993;-1.3e-05 -0.00896170264248081 55.6766643052013 0 -181.3412556811 0 -331.924733815852;-1.25e-05 -0.00896304005647878 55.6860597057402 0 -181.389582490101 0 -331.893786130796;-1.2e-05 -0.00896437724932259 55.6954537322805 0 -181.437904823493 0 -331.862830256589;-1.15e-05 -0.00896571422097927 55.7048463845907 0 -181.486222680084 0 -331.831866193994;-1.1e-05 -0.00896705097141582 55.7142376624389 0 -181.534536058683 0 -331.800893943777;-1.05e-05 -0.00896838750059925 55.7236275655933 0 -181.582844958096 0 -331.769913506701;-1e-05 -0.00896972380849659 55.7330160938224 0 -181.631149377132 0 -331.738924883531;-9.5e-06 -0.00897105989507487 55.7424032468944 0 -181.6794493146 0 -331.70792807503;-9e-06 -0.00897239576030112 55.7517890245777 0 -181.727744769306 0 -331.676923081965;-8.5e-06 -0.00897373140414237 55.7611734266408 0 -181.77603574006 0 -331.645909905099;-8e-06 -0.00897506682656568 55.7705564528521 0 -181.824322225671 0 -331.614888545199;-7.5e-06 -0.00897640202753809 55.77993810298 0 -181.872604224946 0 -331.583859003029;-7e-06 -0.00897773700702667 55.7893183767932 0 -181.920881736694 0 -331.552821279355;-6.5e-06 -0.00897907176499845 55.7986972740601 0 -181.969154759724 0 -331.521775374944;-6e-06 -0.00898040630142053 55.8080747945493 0 -182.017423292846 0 -331.49072129056;-5.5e-06 -0.00898174061625996 55.8174509380295 0 -182.065687334868 0 -331.459659026971;-5e-06 -0.00898307470948382 55.8268257042693 0 -182.113946884598 0 -331.428588584943;-4.5e-06 -0.0089844085810592 55.8361990930374 0 -182.162201940848 0 -331.397509965242;-4e-06 -0.00898574223095319 55.8455711041025 -0.623816098261882 -182.210452502425 0 -331.366423168635;-3.5e-06 -0.00898707565913287 55.8549417372333 -0.623940259551863 -182.25869856814 0 -331.33532819589;-3e-06 -0.00898840886556535 55.8643109921988 -0.624064405446735 -182.306940136801 0 -331.304225047773;-2.5e-06 -0.00898974185021773 55.8736788687676 -0.624188535943435 -182.355177207219 -74.773659636364 -331.273113725052;-2e-06 -0.00899107461305712 55.8830453667086 -0.6243126510389 -182.403409778203 -74.7635329287976 -331.241994228494;-1.5e-06 -0.00899240715405064 55.8924104857907 -0.624436750730068 -182.451637848564 -74.753404376515 -331.210866558868;-1e-06 -0.0089937394731654 55.901774225783 -0.624560835013877 -182.499861417111 -74.743273979766 -331.179730716941;-5e-07 -0.00899507157036854 55.9111365864542 -0.624684903887265 -182.548080482654 -74.7331417388006 -331.148586703482]  x5=1.73744313395484e-05  V1=ones(3,3)  V2=ones(3,3)  I1=ones(3,3)  I2=ones(3,3)  nHarmo=1  Measurements=None  Decoupling=off  VsMag0=0  VrMag0=0  VsAngle0=0  VrAngle0=0  IsMag0=0  IrMag0=0  IsAngle0=0  IrAngle0=0
      settings: LibrarySourceBlock=sps_lib/Power Grid Elements/Distributed Parameters Line
  Ground{1..4} (4 alike) : spsGroundLib/Ground  LConnTagsString=a
  Rcs*1 : spsSeriesRLCBranchLib/Series RLC Branch  LConnTagsString=__new0  RConnTagsString=__new0  BranchType=R  Resistance=-Rg_matrix(1,2)*2  Inductance=1e-3  SetiL0=off  InitialCurrent=0  Capacitance=Rg_matrix(1,2)*2  Setx0=off  InitialVoltage=0  Measurements=None
  Rcs*2 : spsSeriesRLCBranchLib/Series RLC Branch  LConnTagsString=__new0  RConnTagsString=__new0  BranchType=R  Resistance=-Rg_matrix(1,2)*2  Inductance=1e-3  SetiL0=off  InitialCurrent=0  Capacitance=Rg_matrix(1,2)*2  Setx0=off  InitialVoltage=0  Measurements=None
  Rgsg1/1 : spsSeriesRLCBranchLib/Series RLC Branch  LConnTagsString=__new0  RConnTagsString=__new0  BranchType=R  Resistance=(Rg_matrix(4,4)+Rg_matrix(3,4))*2  Inductance=1e-3  SetiL0=off  InitialCurrent=0  Capacitance=Rg_matrix(1,2)*2  Setx0=off  InitialVoltage=0  Measurements=None
  Rgsg1/2 : spsSeriesRLCBranchLib/Series RLC Branch  LConnTagsString=__new0  RConnTagsString=__new0  BranchType=R  Resistance=(Rg_matrix(2,2)+Rg_matrix(1,2))*2  Inductance=1e-3  SetiL0=off  InitialCurrent=0  Capacitance=Rg_matrix(1,2)*2  Setx0=off  InitialVoltage=0  Measurements=None
  Rgsg1/3 : spsSeriesRLCBranchLib/Series RLC Branch  LConnTagsString=__new0  RConnTagsString=__new0  BranchType=R  Resistance=(Rg_matrix(4,4)+Rg_matrix(3,4))*2  Inductance=1e-3  SetiL0=off  InitialCurrent=0  Capacitance=Rg_matrix(1,2)*2  Setx0=off  InitialVoltage=0  Measurements=None
  Rgsg1/4 : spsSeriesRLCBranchLib/Series RLC Branch  LConnTagsString=__new0  RConnTagsString=__new0  BranchType=R  Resistance=(Rg_matrix(2,2)+Rg_matrix(1,2))*2  Inductance=1e-3  SetiL0=off  InitialCurrent=0  Capacitance=Rg_matrix(1,2)*2  Setx0=off  InitialVoltage=0  Measurements=None
  Rsg*1 : spsSeriesRLCBranchLib/Series RLC Branch  LConnTagsString=__new0  RConnTagsString=__new0  BranchType=R  Resistance=(Rg_matrix(6,6)+Rg_matrix(5,6))*2  Inductance=1e-3  SetiL0=off  InitialCurrent=0  Capacitance=Rg_matrix(1,2)*2  Setx0=off  InitialVoltage=0  Measurements=None
  Rsg*2 : spsSeriesRLCBranchLib/Series RLC Branch  LConnTagsString=__new0  RConnTagsString=__new0  BranchType=R  Resistance=(Rg_matrix(6,6)+Rg_matrix(5,6))*2  Inductance=1e-3  SetiL0=off  InitialCurrent=0  Capacitance=Rg_matrix(1,2)*2  Setx0=off  InitialVoltage=0  Measurements=None
  A : PMIOPort  Side=Left
  B : PMIOPort  Port=2  Side=Left
  C : PMIOPort  Port=3  Side=Left
  a : PMIOPort  Port=4  Side=Right
  b : PMIOPort  Port=5  Side=Right
  c : PMIOPort  Port=6  Side=Right
  connections:
  c/RConn1 -- Ccs3/1/RConn1 -- DPL/RConn5
  b/RConn1 -- Ccs2/1/RConn1 -- DPL/RConn3
  a/RConn1 -- DPL/RConn1 -- Rcs*1/RConn1
  Ground4/LConn1 -- DPL/RConn6 -- Ccs3/1/LConn1 -- Rsg*1/LConn1 -- Rcs*1/LConn1 -- Rgsg1/4/LConn1 -- DPL/RConn2 -- DPL/RConn4 -- Ccs2/1/LConn1 -- Rgsg1/3/LConn1
  Ground1/LConn1 -- Rgsg1/4/RConn1 -- Rsg*1/RConn1 -- Rgsg1/3/RConn1
  Ground3/LConn1 -- Ccs3/3/LConn1 -- Rsg*2/LConn1 -- DPL/LConn6 -- Rgsg1/1/LConn1 -- Ccs2/3/LConn1 -- DPL/LConn4 -- Rgsg1/2/LConn1 -- Rcs*2/LConn1 -- DPL/LConn2
  Ground2/LConn1 -- Rgsg1/1/RConn1 -- Rsg*2/RConn1 -- Rgsg1/2/RConn1
  Ccs3/3/RConn1 -- DPL/LConn5 -- C/RConn1
  Ccs2/3/RConn1 -- DPL/LConn3 -- B/RConn1
  Rcs*2/RConn1 -- DPL/LConn1 -- A/RConn1

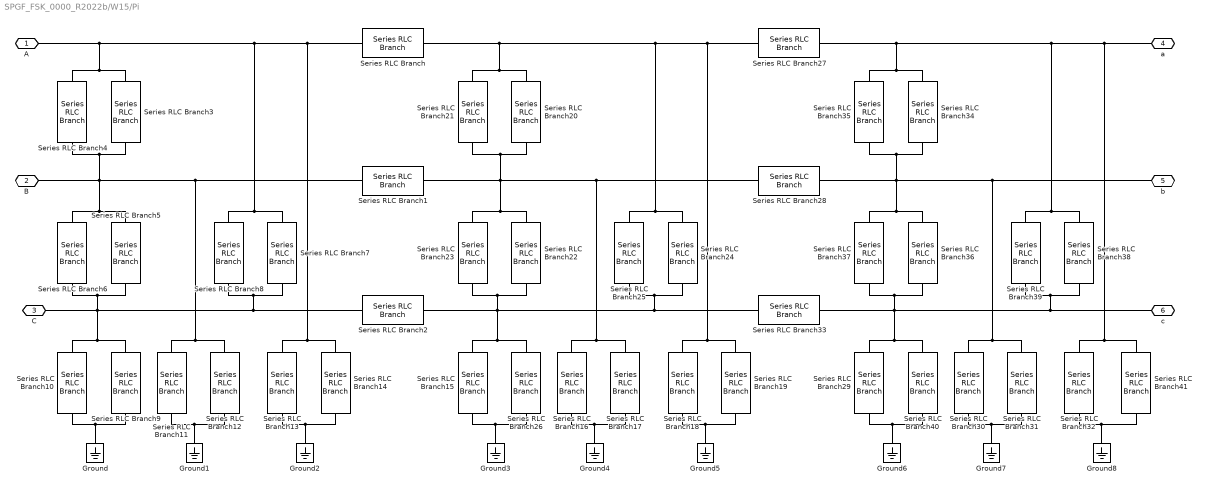
== system SPGF_FSK_0000_R2022b/W15/Pi ==
  Ground{,1..8} (9 alike) : spsGroundLib/Ground  LConnTagsString=a
  Series RLC Branch{,1..2,27..28,33} (6 alike) : spsSeriesRLCBranchLib/Series RLC Branch  LConnTagsString=__new0  RConnTagsString=__new0  BranchType=RL  Resistance=R/2  Inductance=L/2  SetiL0=off  InitialCurrent=0  Capacitance=1e-6  Setx0=off  InitialVoltage=0  Measurements=None
  Series RLC Branch{10..11,13,29..30,32} (6 alike) : spsSeriesRLCBranchLib/Series RLC Branch  LConnTagsString=__new0  RConnTagsString=__new0  BranchType=R  Resistance=Rfg*4  Inductance=L/2  SetiL0=off  InitialCurrent=0  Capacitance=1e-6  Setx0=off  InitialVoltage=0  Measurements=None
  Series RLC Branch{9,12,14,31,40..41} (6 alike) : spsSeriesRLCBranchLib/Series RLC Branch  LConnTagsString=__new0  RConnTagsString=__new0  BranchType=C  Resistance=R/2  Inductance=L/2  SetiL0=off  InitialCurrent=0  Capacitance=Cfg*0.25  Setx0=off  InitialVoltage=0  Measurements=None
  Series RLC Branch15 : spsSeriesRLCBranchLib/Series RLC Branch  LConnTagsString=__new0  RConnTagsString=__new0  BranchType=R  Resistance=Rfg*2  Inductance=L/2  SetiL0=off  InitialCurrent=0  Capacitance=1e-6  Setx0=off  InitialVoltage=0  Measurements=None
  Series RLC Branch16 : spsSeriesRLCBranchLib/Series RLC Branch  LConnTagsString=__new0  RConnTagsString=__new0  BranchType=R  Resistance=Rfg*2  Inductance=L/2  SetiL0=off  InitialCurrent=0  Capacitance=1e-6  Setx0=off  InitialVoltage=0  Measurements=None
  Series RLC Branch17 : spsSeriesRLCBranchLib/Series RLC Branch  LConnTagsString=__new0  RConnTagsString=__new0  BranchType=C  Resistance=R/2  Inductance=L/2  SetiL0=off  InitialCurrent=0  Capacitance=Cfg*0.5  Setx0=off  InitialVoltage=0  Measurements=None
  Series RLC Branch18 : spsSeriesRLCBranchLib/Series RLC Branch  LConnTagsString=__new0  RConnTagsString=__new0  BranchType=R  Resistance=Rfg*2  Inductance=L/2  SetiL0=off  InitialCurrent=0  Capacitance=1e-6  Setx0=off  InitialVoltage=0  Measurements=None
  Series RLC Branch19 : spsSeriesRLCBranchLib/Series RLC Branch  LConnTagsString=__new0  RConnTagsString=__new0  BranchType=C  Resistance=R/2  Inductance=L/2  SetiL0=off  InitialCurrent=0  Capacitance=Cfg*0.5  Setx0=off  InitialVoltage=0  Measurements=None
  Series RLC Branch20 : spsSeriesRLCBranchLib/Series RLC Branch  LConnTagsString=__new0  RConnTagsString=__new0  BranchType=C  Resistance=R/2  Inductance=L/2  SetiL0=off  InitialCurrent=0  Capacitance=Cmf*0.5  Setx0=off  InitialVoltage=0  Measurements=None
  Series RLC Branch21 : spsSeriesRLCBranchLib/Series RLC Branch  LConnTagsString=__new0  RConnTagsString=__new0  BranchType=R  Resistance=Rmf*2  Inductance=L/2  SetiL0=off  InitialCurrent=0  Capacitance=1e-6  Setx0=off  InitialVoltage=0  Measurements=None
  Series RLC Branch22 : spsSeriesRLCBranchLib/Series RLC Branch  LConnTagsString=__new0  RConnTagsString=__new0  BranchType=C  Resistance=R/2  Inductance=L/2  SetiL0=off  InitialCurrent=0  Capacitance=Cmf*0.5  Setx0=off  InitialVoltage=0  Measurements=None
  Series RLC Branch23 : spsSeriesRLCBranchLib/Series RLC Branch  LConnTagsString=__new0  RConnTagsString=__new0  BranchType=R  Resistance=Rmf*2  Inductance=L/2  SetiL0=off  InitialCurrent=0  Capacitance=1e-6  Setx0=off  InitialVoltage=0  Measurements=None
  Series RLC Branch24 : spsSeriesRLCBranchLib/Series RLC Branch  LConnTagsString=__new0  RConnTagsString=__new0  BranchType=C  Resistance=R/2  Inductance=L/2  SetiL0=off  InitialCurrent=0  Capacitance=Cmf*0.5  Setx0=off  InitialVoltage=0  Measurements=None
  Series RLC Branch25 : spsSeriesRLCBranchLib/Series RLC Branch  LConnTagsString=__new0  RConnTagsString=__new0  BranchType=R  Resistance=Rmf*2  Inductance=L/2  SetiL0=off  InitialCurrent=0  Capacitance=1e-6  Setx0=off  InitialVoltage=0  Measurements=None
  Series RLC Branch26 : spsSeriesRLCBranchLib/Series RLC Branch  LConnTagsString=__new0  RConnTagsString=__new0  BranchType=C  Resistance=R/2  Inductance=L/2  SetiL0=off  InitialCurrent=0  Capacitance=Cfg*0.5  Setx0=off  InitialVoltage=0  Measurements=None
  Series RLC Branch{3,5,7,34,36,38} (6 alike) : spsSeriesRLCBranchLib/Series RLC Branch  LConnTagsString=__new0  RConnTagsString=__new0  BranchType=C  Resistance=R/2  Inductance=L/2  SetiL0=off  InitialCurrent=0  Capacitance=Cmf*0.25  Setx0=off  InitialVoltage=0  Measurements=None
  Series RLC Branch{4,6,8,35,37,39} (6 alike) : spsSeriesRLCBranchLib/Series RLC Branch  LConnTagsString=__new0  RConnTagsString=__new0  BranchType=R  Resistance=Rmf*4  Inductance=L/2  SetiL0=off  InitialCurrent=0  Capacitance=1e-6  Setx0=off  InitialVoltage=0  Measurements=None
  A : PMIOPort  Side=Left
  B : PMIOPort  Port=2  Side=Left
  C : PMIOPort  Port=3  Side=Left
  a : PMIOPort  Port=4  Side=Right
  b : PMIOPort  Port=5  Side=Right
  c : PMIOPort  Port=6  Side=Right
  connections:
  Series RLC Branch12/LConn1 -- Series RLC Branch11/LConn1 -- Series RLC Branch5/LConn1 -- Series RLC Branch6/LConn1 -- B/RConn1 -- Series RLC Branch4/RConn1 -- Series RLC Branch3/RConn1 -- Series RLC Branch1/LConn1
  Series RLC Branch13/LConn1 -- A/RConn1 -- Series RLC Branch4/LConn1 -- Series RLC Branch3/LConn1 -- Series RLC Branch7/LConn1 -- Series RLC Branch8/LConn1 -- Series RLC Branch/LConn1 -- Series RLC Branch14/LConn1
  Series RLC Branch9/LConn1 -- Series RLC Branch2/LConn1 -- Series RLC Branch8/RConn1 -- Series RLC Branch7/RConn1 -- C/RConn1 -- Series RLC Branch5/RConn1 -- Series RLC Branch6/RConn1 -- Series RLC Branch10/LConn1
  Series RLC Branch9/RConn1 -- Ground/LConn1 -- Series RLC Branch10/RConn1
  Series RLC Branch12/RConn1 -- Series RLC Branch11/RConn1 -- Ground1/LConn1
  Series RLC Branch13/RConn1 -- Series RLC Branch14/RConn1 -- Ground2/LConn1
  Series RLC Branch17/LConn1 -- Series RLC Branch16/LConn1 -- Series RLC Branch28/LConn1 -- Series RLC Branch1/RConn1 -- Series RLC Branch23/LConn1 -- Series RLC Branch22/LConn1 -- Series RLC Branch20/RConn1 -- Series RLC Branch21/RConn1
  Series RLC Branch21/LConn1 -- Series RLC Branch20/LConn1 -- Series RLC Branch/RConn1 -- Series RLC Branch27/LConn1 -- Series RLC Branch19/LConn1 -- Series RLC Branch18/LConn1 -- Series RLC Branch24/LConn1 -- Series RLC Branch25/LConn1
  Series RLC Branch26/LConn1 -- Series RLC Branch15/LConn1 -- Series RLC Branch2/RConn1 -- Series RLC Branch33/LConn1 -- Series RLC Branch25/RConn1 -- Series RLC Branch24/RConn1 -- Series RLC Branch22/RConn1 -- Series RLC Branch23/RConn1
  Series RLC Branch26/RConn1 -- Series RLC Branch15/RConn1 -- Ground3/LConn1
  Ground4/LConn1 -- Series RLC Branch17/RConn1 -- Series RLC Branch16/RConn1
  Ground5/LConn1 -- Series RLC Branch18/RConn1 -- Series RLC Branch19/RConn1
  Series RLC Branch31/LConn1 -- b/RConn1 -- Series RLC Branch35/RConn1 -- Series RLC Branch34/RConn1 -- Series RLC Branch36/LConn1 -- Series RLC Branch37/LConn1 -- Series RLC Branch28/RConn1 -- Series RLC Branch30/LConn1
  Series RLC Branch34/LConn1 -- a/RConn1 -- Series RLC Branch41/LConn1 -- Series RLC Branch32/LConn1 -- Series RLC Branch38/LConn1 -- Series RLC Branch39/LConn1 -- Series RLC Branch27/RConn1 -- Series RLC Branch35/LConn1
  Series RLC Branch29/LConn1 -- Series RLC Branch36/RConn1 -- Series RLC Branch37/RConn1 -- c/RConn1 -- Series RLC Branch39/RConn1 -- Series RLC Branch38/RConn1 -- Series RLC Branch33/RConn1 -- Series RLC Branch40/LConn1
  Series RLC Branch29/RConn1 -- Series RLC Branch40/RConn1 -- Ground6/LConn1
  Series RLC Branch31/RConn1 -- Series RLC Branch30/RConn1 -- Ground7/LConn1
  Series RLC Branch32/RConn1 -- Series RLC Branch41/RConn1 -- Ground8/LConn1

== system SPGF_FSK_0000_R2022b/W15/Q ==
  breaker : Subsystem  Commented=on  mask{SwitchA=off, SwitchB=off, SwitchC=off, InitialStatus=[1 1 1], BreakerResistance=0.0001, SnubberResistance=1e6, SnubberCapacitance=inf, TransitionTimes=[0.5 0.7], ShiftTimes=[0 0 0]}
      mask prompts: SwitchA "Switching of phase A"; SwitchB "Switching of phase B"; SwitchC "Switching of phase C"; InitialStatus "Initial status of phase breaker [A, B, C]"; BreakerResistance "Breaker resistance Ron (ohms) :"; SnubberResistance "Snubbers resistance Rp (ohms) :"; SnubberCapacitance "Snubbers capacitance Cp (F) :"; TransitionTimes "Transition times (s) :"; ShiftTimes "Time differences for switch [tA, tB, tC] (s) :"
      mask init: same as SPGF_FSK_0000_R2022b/Feed/Q/breaker
      mask Display:
      | % port_label('input',1,'Iabc');
      | 
      | port_label('lconn',1,'A');
      | port_label('lconn',2,'B');
      | port_label('lconn',3,'C');
      | 
      | port_label('rconn',1,'a');
      | port_label('rconn',2,'b');
      | port_label('rconn',3,'c');
      | 
      | disp('   Q    ');
  meas : Subsystem
  shunt : Subsystem
  A : PMIOPort  Side=Right
  B : PMIOPort  Port=2  Side=Right
  C : PMIOPort  Port=3  Side=Right
  a : PMIOPort  Port=4  Side=Left
  b : PMIOPort  Port=5  Side=Left
  c : PMIOPort  Port=6  Side=Left
  connections:
  shunt/LConn3 -- C/RConn1 -- breaker/LConn3
  shunt/LConn2 -- B/RConn1 -- breaker/LConn2
  A/RConn1 -- shunt/LConn1 -- breaker/LConn1
  meas/RConn1 -- a/RConn1
  meas/RConn2 -- b/RConn1
  meas/RConn3 -- c/RConn1
  meas/LConn3 -- breaker/RConn3 -- shunt/RConn3
  meas/LConn2 -- breaker/RConn2 -- shunt/RConn2
  meas/LConn1 -- breaker/RConn1 -- shunt/RConn1
